simulink model "pr523_am_dsb_tc_envelope_detector"  (R2018b)
settings: Solver=VariableStepAuto  StartTime=0.0  StopTime=100*time_span  RelTol=1e-3  EnableMultiTasking=on
PreLoadFcn:
  | pr52setup;
values from neighbouring files (symbols this model uses):
  fs = 500e3    (= 500000)    [pr52setup.m]
undefined symbols (not defined in the file or in its folder): bband1, bband2, bband3, bband4, carrier, single
libraries: dspsrcs4 x6, dspmlti4 x2
CloseFcn:
  | clear all;
settings Model: Creator=GRIHA  LastModifiedBy=Григорий Фокин
settings DataIOCC: LimitDataPoints=on
settings OptimizationCC: LifeSpan=inf
settings DebuggingCC: AllowSymbolicDim=off  SFUnexpectedBacktrackingDiag=warning  SFNoUnconditionalDefaultTransitionDiag=warning  SFExecutionAtInitializationDiag=none
settings ModelReferenceCC: PropagateSignalLabelsOutOfModel=off
settings SFSimCC: SimUseLocalCustomCode=off
settings RTWCC: RTWUseLocalCustomCode=off
settings CodeAppCC: StateflowObjectComments=on
settings GRTTargetCC: TargetLangStandard=C89/C90 (ANSI)
settings ConfigComp: CovMetricSettings=dw  CovHtmlReporting=on  CovSaveCumulativeToWorkspaceVar=on  CovSaveSingleToWorkspaceVar=on  CovExternalEMLEnable=off

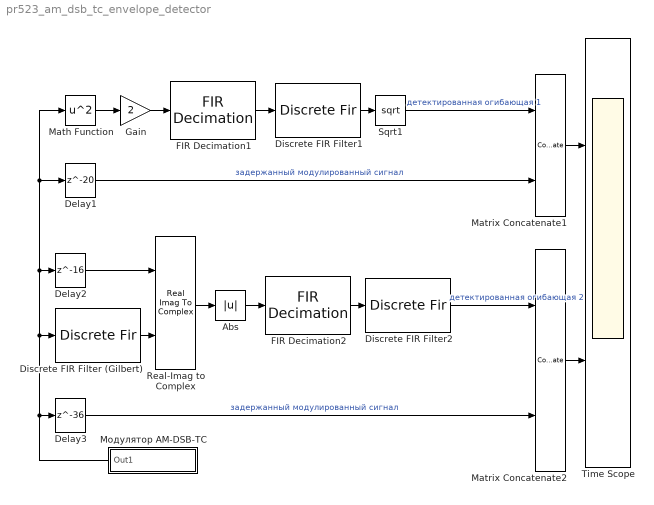
== system pr523_am_dsb_tc_envelope_detector ==
  Abs : Abs
  Delay1 : Delay  DelayLength=20  InitialCondition=0
  Delay2 : Delay  DelayLength=16  InitialCondition=0
  Delay3 : Delay  DelayLength=36  InitialCondition=0
  Discrete FIR Filter (Gilbert) : DiscreteFir  Coefficients=firpm(32, [0.1 0.9], [1 1], 'hilbert')  InputProcessing=Columns as channels (frame based)
  Discrete FIR Filter1 : DiscreteFir  Coefficients=firpm(20, [0 0.03 0.1 1], [1 1 0 0])  InputProcessing=Columns as channels (frame based)
  Discrete FIR Filter2 : DiscreteFir  Coefficients=firpm(20, [0 0.03 0.1 1], [1 1 0 0])  InputProcessing=Columns as channels (frame based)
  FIR Decimation1 : dspmlti4/FIR Decimation  FilterSource=Dialog parameters  h=firpm(20, [0 0.03 0.1 1], [1 1 0 0])  D=2  filtStruct=Direct form  FilterObject=FDECIM  InputProcessing=Columns as channels (frame based)  framing=Allow multirate processing  inputOffset=0  outputBufInitCond=0  roundingMode=Floor  overflowMode=off  firstCoeffDataTypeStr=Inherit: Same word length as input  firstCoeffMin=[]  firstCoeffMax=[]  firstCoeffLastDataTypeStr=Inherit: Same word length as input  outputDataTypeStr=Inherit: Same as accumulator  outputMin=[]  outputMax=[]  outputLastDataTypeStr=Inherit: Same as accumulator
  FIR Decimation2 : dspmlti4/FIR Decimation  FilterSource=Dialog parameters  h=firpm(20, [0 0.03 0.1 1], [1 1 0 0])  D=2  filtStruct=Direct form  FilterObject=FDECIM  InputProcessing=Columns as channels (frame based)  framing=Allow multirate processing  inputOffset=0  outputBufInitCond=0  roundingMode=Floor  overflowMode=off  firstCoeffDataTypeStr=Inherit: Same word length as input  firstCoeffMin=[]  firstCoeffMax=[]  firstCoeffLastDataTypeStr=Inherit: Same word length as input  outputDataTypeStr=Inherit: Same as accumulator  outputMin=[]  outputMax=[]  outputLastDataTypeStr=Inherit: Same as accumulator
  Gain : Gain  Gain=2
  Math Function : Math  Operator=square  SaturateOnIntegerOverflow=on
  Matrix Concatenate1 : Concatenate  Mode=Multidimensional array  ConcatenateDimension=2
  Matrix Concatenate2 : Concatenate  Mode=Multidimensional array  ConcatenateDimension=2
  Real-Imag to Complex : RealImagToComplex
  Sqrt1 : Sqrt  SaturateOnIntegerOverflow=on
  Time Scope : Scope  NumInputPorts=2
  Модулятор AM-DSB-TC : Subsystem
  wires:
  Math Function/1 -> Gain/1
  Gain/1 -> FIR Decimation1/1
  FIR Decimation1/1 -> Discrete FIR Filter1/1
  Discrete FIR Filter1/1 -> Sqrt1/1
  Sqrt1/1 -> Matrix Concatenate1/1  "детектированная огибающая 1"
  Delay1/1 -> Matrix Concatenate1/2  "задержанный модулированный сигнал"
  Matrix Concatenate1/1 -> Time Scope/1
  Discrete FIR Filter (Gilbert)/1 -> Real-Imag to Complex/2
  Delay2/1 -> Real-Imag to Complex/1
  Real-Imag to Complex/1 -> Abs/1
  Abs/1 -> FIR Decimation2/1
  FIR Decimation2/1 -> Discrete FIR Filter2/1
  Discrete FIR Filter2/1 -> Matrix Concatenate2/1  "детектированная огибающая 2"
  Delay3/1 -> Matrix Concatenate2/2  "задержанный модулированный сигнал"
  Matrix Concatenate2/1 -> Time Scope/2
  Модулятор AM-DSB-TC/1(Out1) -> Math Function/1, Delay1/1, Delay2/1, Discrete FIR Filter (Gilbert)/1, Delay3/1

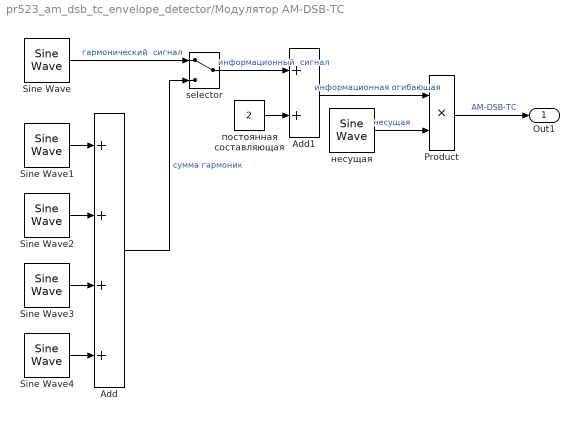
== system pr523_am_dsb_tc_envelope_detector/Модулятор AM-DSB-TC ==
  Add : Sum  Inputs=++++
  Add1 : Sum
  Product : Product
  Sine Wave : dspsrcs4/Sine Wave  Amplitude=single.Ai  Frequency=single.fi  Phase=single.ph  SampleMode=Discrete  OutComplex=Real  CompMethod=Trigonometric fcn  TableSize=Speed  SampleTime=1/fs  SamplesPerFrame=1  ResetState=Restart at time zero  OutputFrames=off  dataType=double  wordLen=16  udDataType=sfix(16)  fracBitsMode=Best precision  numFracBits=15  OutDataTypeStr=double  LastOutDataTypeStr=double
  Sine Wave1 : dspsrcs4/Sine Wave  Amplitude=bband1.Ai  Frequency=bband1.fi  Phase=bband1.ph  SampleMode=Discrete  OutComplex=Real  CompMethod=Trigonometric fcn  TableSize=Speed  SampleTime=1/fs  SamplesPerFrame=1  ResetState=Restart at time zero  OutputFrames=off  dataType=double  wordLen=16  udDataType=sfix(16)  fracBitsMode=Best precision  numFracBits=15  OutDataTypeStr=double  LastOutDataTypeStr=double
  Sine Wave2 : dspsrcs4/Sine Wave  Amplitude=bband2.Ai  Frequency=bband2.fi  Phase=bband2.ph  SampleMode=Discrete  OutComplex=Real  CompMethod=Trigonometric fcn  TableSize=Speed  SampleTime=1/fs  SamplesPerFrame=1  ResetState=Restart at time zero  OutputFrames=off  dataType=double  wordLen=16  udDataType=sfix(16)  fracBitsMode=Best precision  numFracBits=15  OutDataTypeStr=double  LastOutDataTypeStr=double
  Sine Wave3 : dspsrcs4/Sine Wave  Amplitude=bband3.Ai  Frequency=bband3.fi  Phase=bband3.ph  SampleMode=Discrete  OutComplex=Real  CompMethod=Trigonometric fcn  TableSize=Speed  SampleTime=1/fs  SamplesPerFrame=1  ResetState=Restart at time zero  OutputFrames=off  dataType=double  wordLen=16  udDataType=sfix(16)  fracBitsMode=Best precision  numFracBits=15  OutDataTypeStr=double  LastOutDataTypeStr=double
  Sine Wave4 : dspsrcs4/Sine Wave  Amplitude=bband4.Ai  Frequency=bband4.fi  Phase=bband4.ph  SampleMode=Discrete  OutComplex=Real  CompMethod=Trigonometric fcn  TableSize=Speed  SampleTime=1/fs  SamplesPerFrame=1  ResetState=Restart at time zero  OutputFrames=off  dataType=double  wordLen=16  udDataType=sfix(16)  fracBitsMode=Best precision  numFracBits=15  OutDataTypeStr=double  LastOutDataTypeStr=double
  selector : ManualSwitch
  несущая : dspsrcs4/Sine Wave  Amplitude=carrier.Ac  Frequency=carrier.fc  Phase=carrier.ph  SampleMode=Discrete  OutComplex=Real  CompMethod=Trigonometric fcn  TableSize=Speed  SampleTime=1/fs  SamplesPerFrame=1  ResetState=Restart at time zero  OutputFrames=off  dataType=double  wordLen=16  udDataType=sfix(16)  fracBitsMode=Best precision  numFracBits=15  OutDataTypeStr=double  LastOutDataTypeStr=double
  постоянная составляющая : Constant  Value=2
  Out1 : Outport
  wires:
  Sine Wave2/1 -> Add/2
  Sine Wave4/1 -> Add/4
  несущая/1 -> Product/2  "несущая"
  selector/1 -> Add1/1  "информационный  сигнал"
  постоянная составляющая/1 -> Add1/2
  Sine Wave1/1 -> Add/1
  Add1/1 -> Product/1  "информационная огибающая"
  Add/1 -> selector/2  "сумма гармоник"
  Sine Wave3/1 -> Add/3
  Sine Wave/1 -> selector/1  "гармонический  сигнал"
  Product/1 -> Out1/1  "AM-DSB-TC"
